simulink model "Example_8_3b"  (R2014a)
settings: Solver=FixedStepDiscrete  SolverMode=SingleTasking  StartTime=0.0  StopTime=20  RelTol=1e-3
InitFcn:
  |  b=[14 37.39 27.24 6.26 12.481 11.6605 ...
  |  -5.7215 -3.8865 .5425];
  | a=[1 .9 .5 .08 .14 .353 -.244 -.289 -.182 -.01 .072];
libraries: dspsrcs4 x1
settings Model: Creator=Lee Edwards  LastModifiedBy=Lee
settings DataIOCC: SignalLoggingSaveFormat=ModelDataLogs  SaveOutput=off  SignalLogging=off  SaveTime=off
settings OptimizationCC: ExpressionDepthLimit=2147483647
settings DebuggingCC: AlgebraicLoopMsg=error  UnderspecifiedInitializationDetection=Classic  SingleTaskRateTransMsg=error  FcnCallInpInsideContextMsg=UseLocalSettings  StateNameClashWarn=warning
settings GRTTargetCC: CombineOutputUpdateFcns=off  GRTInterface=on

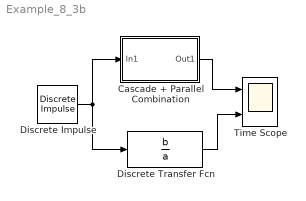
== system Example_8_3b ==
  "Cascade + Parallel Combination " : Subsystem
  Discrete Transfer Fcn : DiscreteTransferFcn  Numerator=b  Denominator=a
  Discrete Impulse : dspsrcs4/Discrete  Impulse  Delay=0  SampleTime=1  FrameSample=1  dataType=double  isSigned=on  wordLen=16  udDataType=sfix(16)  fracBitsMode=Best precision  numFracBits=15  OutDataTypeStr=double  LastOutDataTypeStr=double
  Time Scope : Scope  NumInputPorts=2
      settings: YMin=-30~-30  YMax=30~30  DataFormat=Structure
  wires:
  "Cascade + Parallel Combination "/1(Out1) -> Time Scope/1
  Discrete Transfer Fcn/1 -> Time Scope/2
  Discrete Impulse/1 -> "Cascade + Parallel Combination "/1(In1), Discrete Transfer Fcn/1

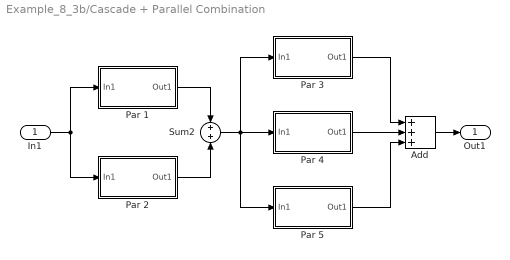
== system Example_8_3b/Cascade + Parallel Combination  ==
  In1 : Inport
  Add : Sum  Inputs=+++
  Par 1 : Subsystem
  Par 2 : Subsystem
  Par 3 : Subsystem
  Par 4 : Subsystem
  Par 5 : Subsystem
  Sum2 : Sum  Inputs=+|+
  Out1 : Outport
  wires:
  Par 2/1(Out1) -> Sum2/2
  Par 1/1(Out1) -> Sum2/1
  In1/1 -> Par 1/1(In1), Par 2/1(In1)
  Sum2/1 -> Par 4/1(In1), Par 3/1(In1), Par 5/1(In1)
  Par 3/1(Out1) -> Add/1
  Par 4/1(Out1) -> Add/2
  Par 5/1(Out1) -> Add/3
  Add/1 -> Out1/1

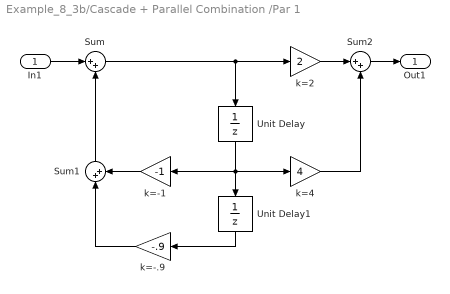
== system Example_8_3b/Cascade + Parallel Combination /Par 1 ==
  In1 : Inport
  Sum : Sum  Inputs=|++
  Sum1 : Sum  Inputs=|++
  Sum2 : Sum  Inputs=|++
  Unit Delay : UnitDelay  SampleTime=-1
  Unit Delay1 : UnitDelay  SampleTime=-1
  k=-.9 : Gain  Gain=-.9
  k=-1 : Gain  Gain=-1
  k=2 : Gain  Gain=2
  k=4 : Gain  Gain=4
  Out1 : Outport
  wires:
  Unit Delay/1 -> Unit Delay1/1, k=-1/1, k=4/1
  Unit Delay1/1 -> k=-.9/1
  k=-1/1 -> Sum1/2
  k=-.9/1 -> Sum1/1
  In1/1 -> Sum/1
  Sum1/1 -> Sum/2
  Sum/1 -> k=2/1, Unit Delay/1
  k=2/1 -> Sum2/1
  k=4/1 -> Sum2/2
  Sum2/1 -> Out1/1

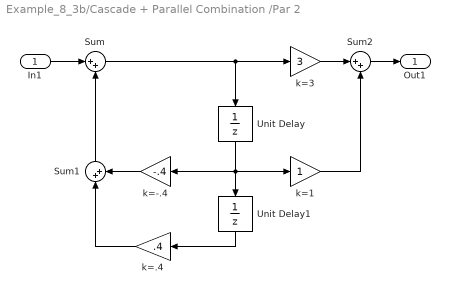
== system Example_8_3b/Cascade + Parallel Combination /Par 2 ==
  In1 : Inport
  Sum : Sum  Inputs=|++
  Sum1 : Sum  Inputs=|++
  Sum2 : Sum  Inputs=|++
  Unit Delay : UnitDelay  SampleTime=-1
  Unit Delay1 : UnitDelay  SampleTime=-1
  k=-.4 : Gain  Gain=-.4
  k=.4 : Gain  Gain=.4
  k=1 : Gain
  k=3 : Gain  Gain=3
  Out1 : Outport
  wires:
  Unit Delay/1 -> Unit Delay1/1, k=-.4/1, k=1/1
  Unit Delay1/1 -> k=.4/1
  k=-.4/1 -> Sum1/2
  k=.4/1 -> Sum1/1
  In1/1 -> Sum/1
  Sum1/1 -> Sum/2
  Sum/1 -> Unit Delay/1, k=3/1
  k=3/1 -> Sum2/1
  k=1/1 -> Sum2/2
  Sum2/1 -> Out1/1

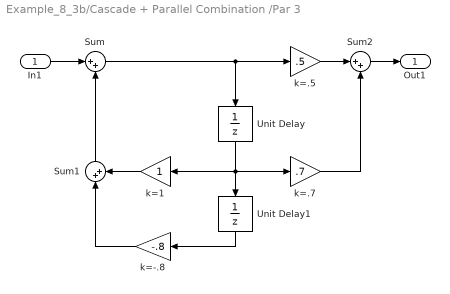
== system Example_8_3b/Cascade + Parallel Combination /Par 3 ==
  In1 : Inport
  Sum : Sum  Inputs=|++
  Sum1 : Sum  Inputs=|++
  Sum2 : Sum  Inputs=|++
  Unit Delay : UnitDelay  SampleTime=-1
  Unit Delay1 : UnitDelay  SampleTime=-1
  k=-.8 : Gain  Gain=-.8
  k=.5 : Gain  Gain=.5
  k=.7 : Gain  Gain=.7
  k=1 : Gain
  Out1 : Outport
  wires:
  Unit Delay/1 -> Unit Delay1/1, k=1/1, k=.7/1
  Unit Delay1/1 -> k=-.8/1
  k=1/1 -> Sum1/2
  k=-.8/1 -> Sum1/1
  In1/1 -> Sum/1
  Sum1/1 -> Sum/2
  Sum/1 -> Unit Delay/1, k=.5/1
  k=.5/1 -> Sum2/1
  k=.7/1 -> Sum2/2
  Sum2/1 -> Out1/1

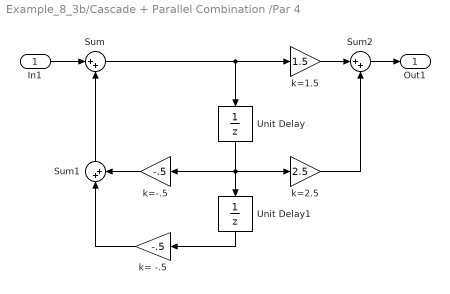
== system Example_8_3b/Cascade + Parallel Combination /Par 4 ==
  In1 : Inport
  Sum : Sum  Inputs=|++
  Sum1 : Sum  Inputs=|++
  Sum2 : Sum  Inputs=|++
  Unit Delay : UnitDelay  SampleTime=-1
  Unit Delay1 : UnitDelay  SampleTime=-1
  k= -.5 : Gain  Gain=-.5
  k=-.5 : Gain  Gain=-.5
  k=1.5 : Gain  Gain=1.5
  k=2.5 : Gain  Gain=2.5
  Out1 : Outport
  wires:
  Unit Delay/1 -> Unit Delay1/1, k=-.5/1, k=2.5/1
  Unit Delay1/1 -> k= -.5/1
  k=-.5/1 -> Sum1/2
  k= -.5/1 -> Sum1/1
  In1/1 -> Sum/1
  Sum1/1 -> Sum/2
  Sum/1 -> Unit Delay/1, k=1.5/1
  k=1.5/1 -> Sum2/1
  k=2.5/1 -> Sum2/2
  Sum2/1 -> Out1/1

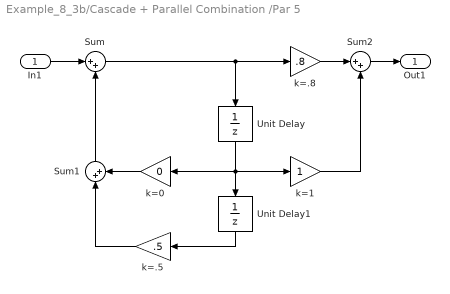
== system Example_8_3b/Cascade + Parallel Combination /Par 5 ==
  In1 : Inport
  Sum : Sum  Inputs=|++
  Sum1 : Sum  Inputs=|++
  Sum2 : Sum  Inputs=|++
  Unit Delay : UnitDelay  SampleTime=-1
  Unit Delay1 : UnitDelay  SampleTime=-1
  k=.5 : Gain  Gain=.5
  k=.8 : Gain  Gain=.8
  k=0 : Gain  Gain=0
  k=1 : Gain
  Out1 : Outport
  wires:
  Unit Delay/1 -> Unit Delay1/1, k=0/1, k=1/1
  Unit Delay1/1 -> k=.5/1
  k=0/1 -> Sum1/2
  k=.5/1 -> Sum1/1
  In1/1 -> Sum/1
  Sum1/1 -> Sum/2
  Sum/1 -> Unit Delay/1, k=.8/1
  k=.8/1 -> Sum2/1
  k=1/1 -> Sum2/2
  Sum2/1 -> Out1/1
